simulink model "d"  (R2018b)
settings: Solver=FixedStepAuto  StartTime=0.0  StopTime=10.68  FixedStep=0.01  RelTol=1e-3
settings Model: Creator=yizha  LastModifiedBy=yizha

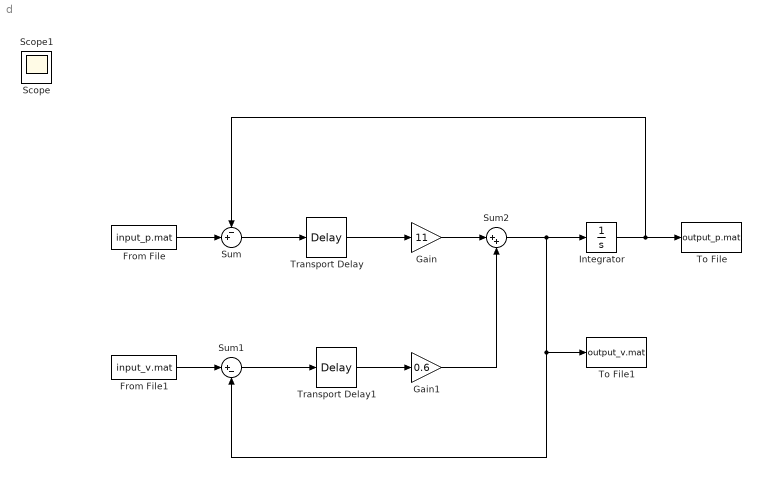
== system d ==
  From File : FromFile  FileName=input_p.mat  SampleTime=0
  From File1 : FromFile  FileName=input_v.mat  SampleTime=0
  Gain : Gain  Gain=11
  Gain1 : Gain  Gain=0.6
  Integrator : Integrator
  Sum : Sum  Inputs=-+|
  Sum1 : Sum  Inputs=|+-
  Sum2 : Sum  Inputs=|++
  To File : ToFile  Filename=output_p.mat
  To File1 : ToFile  Filename=output_v.mat
  Transport Delay : TransportDelay  DelayTime=0.1
  Transport Delay1 : TransportDelay  DelayTime=0.1
  Scope : Scope
  Scope1 : Scope
  wires:
  Sum/1 -> Transport Delay/1
  Transport Delay/1 -> Gain/1
  Integrator/1 -> To File/1, Sum/1
  From File1/1 -> Sum1/1
  Sum1/1 -> Transport Delay1/1
  Transport Delay1/1 -> Gain1/1
  Gain/1 -> Sum2/1
  Sum2/1 -> Integrator/1, To File1/1, Sum1/2
  Gain1/1 -> Sum2/2
  From File/1 -> Sum/2
